simulink model "3.jmavsim_control_smc"  (R2023b)
settings: Solver=FixedStepAuto  StartTime=0.0  StopTime=inf  FixedStep=0.01  RelTol=1e-3  EnableMultiTasking=on
undefined symbols (not defined in the file): dev, Main, pwm_output0
libraries: simulink x19, px4uORBlib x3, sharedtransform x1, px4lib x1
settings Model: ExtModeTrigDuration=10  Creator=UAV2  LastModifiedBy=UAV2
settings SolverCC: PositivePriorityOrder=on
settings OptimizationCC: EnhancedBackFolding=on  PassReuseOutputArgsAs=Individual arguments  ZeroExternalMemoryAtStartup=off  ZeroInternalMemoryAtStartup=off  MaxStackSize=64  OptimizeBlockOrder=speed  DifferentSizesBufferReuse=on  EfficientTunableParamExpr=on
settings DebuggingCC: ParameterTunabilityLossMsg=error
settings HardwareCC: ProdBitPerPointer=32  ProdBitPerSizeT=32  ProdBitPerPtrDiffT=32  ProdLargestAtomicInteger=Long  ProdLargestAtomicFloat=Double  ProdWordSize=32  ProdLongLongMode=on  ProdHWDeviceType=ARM Compatible->ARM Cortex
settings SFSimCC: MATLABDynamicMemAlloc=off  SimTargetLang=C++
settings RTWCC: Description=Embedded Coder  SystemTargetFile=ert.tlc  HardwareBoard=PX4 Host Target  TemplateMakefile=ert_default_tmf  Toolchain=GNU Tools for PX4 Autopilots  PortableWordSizes=on  TargetLang=C++
settings CodeAppCC: ForceParamTrailComments=on  IgnoreCustomStorageClasses=off  OperatorAnnotations=on  SimulinkDataObjDesc=on  SFDataObjDesc=on  InsertBlockDesc=on
settings ERTTargetCC: ExtMode=on  ExtModeTransport=2  ExtModeStaticAlloc=on  ExtModeMexFile=ext_xcp  ExtModeMexArgs='127.0.0.1' 1 17725  ExtModeIntrfLevel=Level2 - Open

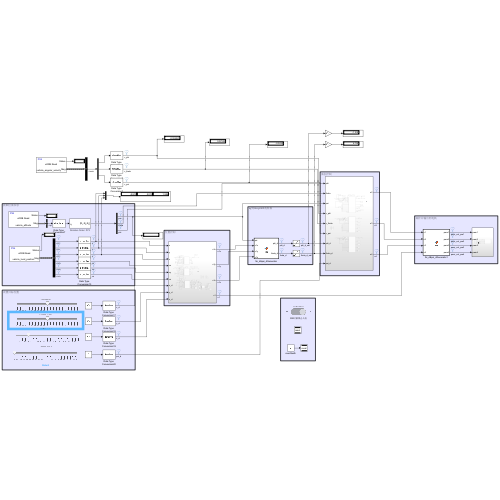
[thumbnail: Simulink's stored preview of the top-level diagram]
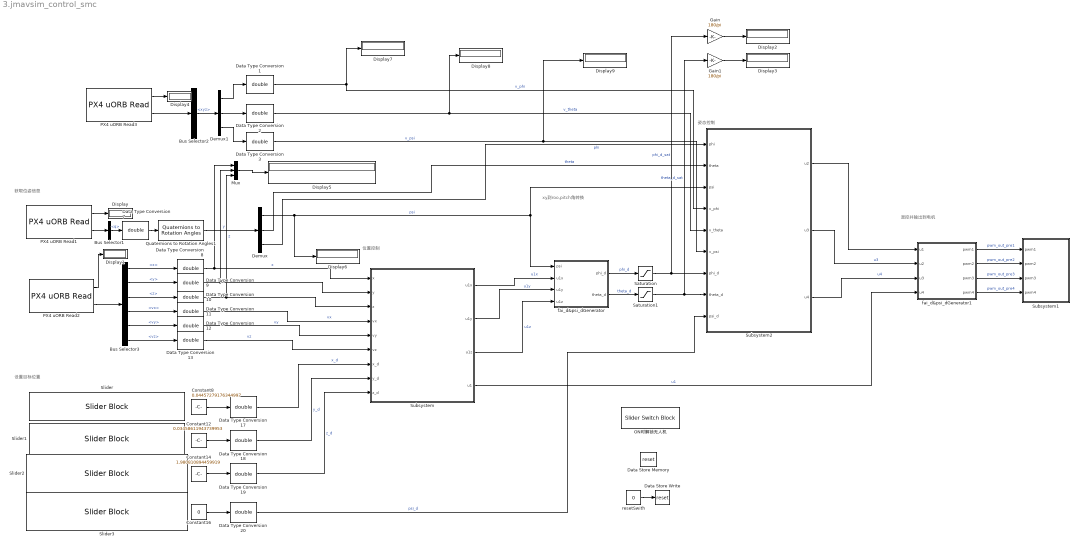
== system 3.jmavsim_control_smc ==
  note: 混控并输出到电机
  note: xy到roo,pitch角转换
  note: 姿态控制
  note: 位置控制
  note: 设置目标位置
  note: 获取位姿信息
  Bus Selector1 : BusSelector  OutputSignals=q
  Bus Selector2 : BusSelector  OutputSignals=xyz
  Bus Selector3 : BusSelector  OutputSignals=x,y,z,vx,vy,vz
  Constant12 : Constant  Value=0.03458611943739953
  Constant14 : Constant  Value=1.980810894459919
  Constant16 : Constant  Value=0
  Constant8 : Constant  Value=0.04457279176344997
  Data Store Memory : DataStoreMemory  DataStoreName=reset  WriteAfterWriteMsg=warning  ShowAdditionalParam=off  OutDataTypeStr=boolean
  Data Store Write : DataStoreWrite  DataStoreName=reset  IndexOptions=Index vector (dialog)  Indices=1  OutputSizes=1
  Data Type Conversion{1..3,7..13,17..20} (14 alike) : DataTypeConversion  OutDataTypeStr=double  SaturateOnIntegerOverflow=off  RndMeth=Floor
  Demux : Demux  Outputs=3
  Demux1 : Demux  Outputs=3
  Display{,1..9} (10 alike) : Display
      Display5 settings: Decimation=3
  Gain : Gain  Gain=180/pi
  Gain1 : Gain  Gain=180/pi
  Mux : Mux  Inputs=3
  ON时解锁无人机 : SliderSwitchBlock  Description=1时解锁无人机
      settings: Values={{'Off', 'On'}, [1 0]}
  PX4 uORB Read1 : px4uORBlib/PX4 uORB Read  uORBTopic=vehicle_attitude  selectInstance=vehicle_attitude_groundtruth  SampleTime=-1  BlockingMode=off  BlockTimeout=1e-3
  PX4 uORB Read2 : px4uORBlib/PX4 uORB Read  uORBTopic=vehicle_local_position  selectInstance=vehicle_local_position_groundtruth  SampleTime=-1  BlockingMode=off  BlockTimeout=1e-3
  PX4 uORB Read3 : px4uORBlib/PX4 uORB Read  uORBTopic=vehicle_angular_velocity  selectInstance=vehicle_angular_velocity  SampleTime=-1  BlockingMode=off  BlockTimeout=1e-3
  Quaternions to Rotation Angles1 : sharedtransform/Quaternions to Rotation Angles  rotationOrder=ZYX  aMode=aMode
  Saturation : Saturate
  Saturation1 : Saturate
  Slider : SliderBlock  ScaleMin=-10  ScaleMax=10
  Slider1 : SliderBlock  ScaleMin=-10  ScaleMax=10
  Slider2 : SliderBlock  ScaleMax=10
  Slider3 : SliderBlock  ScaleMax=2
  Subsystem : Subsystem
  Subsystem1 : Subsystem
  Subsystem2 : Subsystem
  fai_d&psi_dGenerator : MATLAB Function  TreatAsAtomicUnit=on
  fai_d&psi_dGenerator1 : MATLAB Function  TreatAsAtomicUnit=on
  resetSwith : Constant  Value=0  OutDataTypeStr=boolean
  wires:
  Constant8/1 -> Data Type Conversion17/1
  Quaternions to Rotation Angles1/1 -> Demux/1
  PX4 uORB Read1/1 -> Display/1
  PX4 uORB Read1/2 -> Bus Selector1/1
  Bus Selector1/1 -> Data Type Conversion7/1  "<q>"
  Data Type Conversion7/1 -> Quaternions to Rotation Angles1/1
  resetSwith/1 -> Data Store Write/1
  PX4 uORB Read2/2 -> Bus Selector3/1
  Bus Selector3/2 -> Data Type Conversion9/1  "<y>"
  Bus Selector3/3 -> Data Type Conversion10/1  "<z>"
  Bus Selector3/4 -> Data Type Conversion11/1  "<vx>"
  Bus Selector3/5 -> Data Type Conversion12/1  "<vy>"
  Bus Selector3/6 -> Data Type Conversion13/1  "<vz>"
  Bus Selector3/1 -> Data Type Conversion8/1  "<x>"
  PX4 uORB Read2/1 -> Display1/1
  Subsystem/2(u1y) -> fai_d&psi_dGenerator/3(u1y)  "u1y"
  fai_d&psi_dGenerator1/1(pwm1) -> Subsystem1/1(pwm1)  "pwm_out_pre1"
  fai_d&psi_dGenerator1/2(pwm2) -> Subsystem1/2(pwm2)  "pwm_out_pre2"
  fai_d&psi_dGenerator1/3(pwm3) -> Subsystem1/3(pwm3)  "pwm_out_pre3"
  fai_d&psi_dGenerator1/4(pwm4) -> Subsystem1/4(pwm4)  "pwm_out_pre4"
  Demux/1 -> Display6/1, fai_d&psi_dGenerator/1(psi), Subsystem2/3(psi)  "psi"
  Demux/2 -> Subsystem2/2(theta)  "theta"
  Demux/3 -> Subsystem2/1(phi)  "phi"
  Constant12/1 -> Data Type Conversion18/1
  Constant14/1 -> Data Type Conversion19/1
  Constant16/1 -> Data Type Conversion20/1
  Data Type Conversion20/1 -> Subsystem2/9(psi_d)  "psi_d"
  fai_d&psi_dGenerator/1(phi_d) -> Saturation/1  "phi_d"
  fai_d&psi_dGenerator/2(theta_d) -> Saturation1/1  "theta_d"
  Subsystem/3(u1z) -> fai_d&psi_dGenerator/4(u1z)  "u1z"
  Subsystem/4(u1) -> fai_d&psi_dGenerator1/4(u4)  "u1"
  Saturation1/1 -> Subsystem2/8(theta_d), Gain1/1  "theta_d_sat"
  Data Type Conversion8/1 -> Mux/1, Subsystem/1(x)  "x"
  Data Type Conversion9/1 -> Mux/2, Subsystem/2(y)  "y"
  Data Type Conversion10/1 -> Mux/3, Subsystem/3(z)  "z"
  Data Type Conversion12/1 -> Subsystem/5(vy)  "vy"
  Data Type Conversion13/1 -> Subsystem/6(vz)  "vz"
  Data Type Conversion17/1 -> Subsystem/7(x_d)  "x_d"
  Data Type Conversion18/1 -> Subsystem/8(y_d)  "y_d"
  Data Type Conversion19/1 -> Subsystem/9(z_d)  "z_d"
  Data Type Conversion11/1 -> Subsystem/4(vx)  "vx"
  Subsystem/1(u1x) -> fai_d&psi_dGenerator/2(u1x)  "u1x"
  Gain/1 -> Display2/1
  Gain1/1 -> Display3/1
  PX4 uORB Read3/2 -> Bus Selector2/1
  PX4 uORB Read3/1 -> Display4/1
  Data Type Conversion1/1 -> Display7/1, Subsystem2/4(v_phi)  "v_phi"
  Data Type Conversion2/1 -> Display8/1, Subsystem2/5(v_theta)  "v_theta"
  Data Type Conversion3/1 -> Display9/1, Subsystem2/6(v_psi)  "v_psi"
  Mux/1 -> Display5/1
  Bus Selector2/1 -> Demux1/1  "<xyz>"
  Demux1/1 -> Data Type Conversion1/1
  Demux1/2 -> Data Type Conversion2/1
  Demux1/3 -> Data Type Conversion3/1
  Saturation/1 -> Gain/1, Subsystem2/7(phi_d)  "phi_d_sat"
  Subsystem2/3(u4) -> fai_d&psi_dGenerator1/3(u3)  "u4"
  Subsystem2/1(u2) -> fai_d&psi_dGenerator1/1(u1)
  Subsystem2/2(u3) -> fai_d&psi_dGenerator1/2(u2)  "u3"

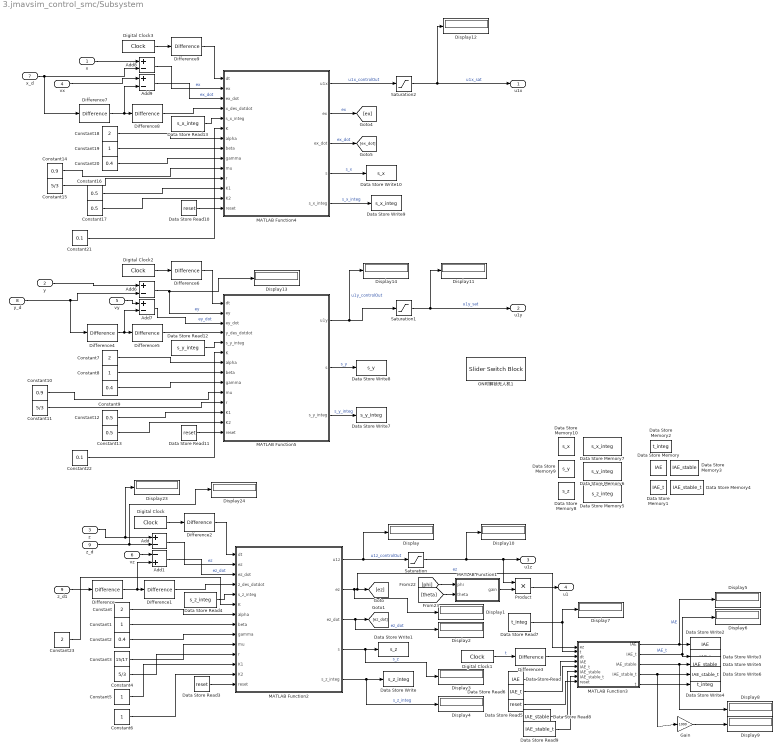
== system 3.jmavsim_control_smc/Subsystem ==
  x : Inport
  y : Inport  Port=2
  z : Inport  Port=3
  vx : Inport  Port=4
  vy : Inport  Port=5
  vz : Inport  Port=6
  x_d : Inport  Port=7
  y_d : Inport  Port=8
  z_d : Inport  Port=9
  Add{,6..9} (5 alike) : Sum  Inputs=+-
  Add1 : Sum  Inputs=-+
  Constant{,7,18,23} (4 alike) : Constant  Value=2
  Constant{1,5..6,8,19} (5 alike) : Constant
  Constant10 : Constant  Value=0.9
  Constant11 : Constant  Value=5/3
  Constant{12..13,16..17} (4 alike) : Constant  Value=0.5
  Constant14 : Constant  Value=0.9
  Constant15 : Constant  Value=5/3
  Constant2 : Constant  Value=0.4
  Constant20 : Constant  Value=0.4
  Constant21 : Constant  Value=0.1
  Constant22 : Constant  Value=0.1
  Constant3 : Constant  Value=15/17
  Constant4 : Constant  Value=5/3
  Constant9 : Constant  Value=0.4
  Data Store Memory : DataStoreMemory  DataStoreName=IAE  WriteAfterWriteMsg=warning  ShowAdditionalParam=off
  Data Store Memory1 : DataStoreMemory  DataStoreName=IAE_t  WriteAfterWriteMsg=warning  ShowAdditionalParam=off
  Data Store Memory10 : DataStoreMemory  DataStoreName=s_x  WriteAfterWriteMsg=warning  ShowAdditionalParam=off  OutDataTypeStr=double
  Data Store Memory2 : DataStoreMemory  DataStoreName=t_integ  WriteAfterWriteMsg=warning  ShowAdditionalParam=off
  Data Store Memory3 : DataStoreMemory  DataStoreName=IAE_stable  WriteAfterWriteMsg=warning  ShowAdditionalParam=off
  Data Store Memory4 : DataStoreMemory  DataStoreName=IAE_stable_t  WriteAfterWriteMsg=warning  ShowAdditionalParam=off
  Data Store Memory5 : DataStoreMemory  DataStoreName=s_z_integ  WriteAfterWriteMsg=warning  ShowAdditionalParam=off  OutDataTypeStr=double
  Data Store Memory6 : DataStoreMemory  DataStoreName=s_y_integ  WriteAfterWriteMsg=warning  ShowAdditionalParam=off  OutDataTypeStr=double
  Data Store Memory7 : DataStoreMemory  DataStoreName=s_x_integ  WriteAfterWriteMsg=warning  ShowAdditionalParam=off  OutDataTypeStr=double
  Data Store Memory8 : DataStoreMemory  DataStoreName=s_z  WriteAfterWriteMsg=warning  ShowAdditionalParam=off  OutDataTypeStr=double
  Data Store Memory9 : DataStoreMemory  DataStoreName=s_y  WriteAfterWriteMsg=warning  ShowAdditionalParam=off  OutDataTypeStr=double
  Data Store Read : DataStoreRead  DataStoreName=IAE  IndexOptions=Index vector (dialog)  Indices=1  OutputSizes=1
  Data Store Read{3,5,10..11} (4 alike) : DataStoreRead  DataStoreName=reset  IndexOptions=Index vector (dialog)  Indices=1  OutputSizes=1
  Data Store Read12 : DataStoreRead  DataStoreName=s_y_integ  IndexOptions=Index vector (dialog)  Indices=1  OutputSizes=1
  Data Store Read13 : DataStoreRead  DataStoreName=s_x_integ  IndexOptions=Index vector (dialog)  Indices=1  OutputSizes=1
  Data Store Read4 : DataStoreRead  DataStoreName=s_z_integ  IndexOptions=Index vector (dialog)  Indices=1  OutputSizes=1
  Data Store Read6 : DataStoreRead  DataStoreName=IAE_t  IndexOptions=Index vector (dialog)  Indices=1  OutputSizes=1
  Data Store Read7 : DataStoreRead  DataStoreName=t_integ  IndexOptions=Index vector (dialog)  Indices=1  OutputSizes=1
  Data Store Read8 : DataStoreRead  DataStoreName=IAE_stable  IndexOptions=Index vector (dialog)  Indices=1  OutputSizes=1
  Data Store Read9 : DataStoreRead  DataStoreName=IAE_stable_t  IndexOptions=Index vector (dialog)  Indices=1  OutputSizes=1
  Data Store Write : DataStoreWrite  DataStoreName=s_z_integ  IndexOptions=Index vector (dialog)  Indices=1  OutputSizes=1
  Data Store Write1 : DataStoreWrite  DataStoreName=s_z  IndexOptions=Index vector (dialog)  Indices=1  OutputSizes=1
  Data Store Write10 : DataStoreWrite  DataStoreName=s_x  IndexOptions=Index vector (dialog)  Indices=1  OutputSizes=1
  Data Store Write2 : DataStoreWrite  DataStoreName=IAE  IndexOptions=Index vector (dialog)  Indices=1  OutputSizes=1
  Data Store Write3 : DataStoreWrite  DataStoreName=IAE_t  IndexOptions=Index vector (dialog)  Indices=1  OutputSizes=1
  Data Store Write4 : DataStoreWrite  DataStoreName=t_integ  IndexOptions=Index vector (dialog)  Indices=1  OutputSizes=1
  Data Store Write5 : DataStoreWrite  DataStoreName=IAE_stable  IndexOptions=Index vector (dialog)  Indices=1  OutputSizes=1
  Data Store Write6 : DataStoreWrite  DataStoreName=IAE_stable_t  IndexOptions=Index vector (dialog)  Indices=1  OutputSizes=1
  Data Store Write7 : DataStoreWrite  DataStoreName=s_y_integ  IndexOptions=Index vector (dialog)  Indices=1  OutputSizes=1
  Data Store Write8 : DataStoreWrite  DataStoreName=s_y  IndexOptions=Index vector (dialog)  Indices=1  OutputSizes=1
  Data Store Write9 : DataStoreWrite  DataStoreName=s_x_integ  IndexOptions=Index vector (dialog)  Indices=1  OutputSizes=1
  Difference{,1..9} (10 alike) : simulink/Discrete/Difference  ICPrevInput=0.0  OutMin=[]  OutMax=[]  OutDataType=fixdt(1, 16)  OutScaling=2^-10  DoSatur=off
  Digital Clock{,1..3} (4 alike) : DigitalClock  SampleTime=0.01
  Display{,1..14,23..24} (17 alike) : Display
  Gain : Gain  Gain=1000
  MATLAB Function1 : MATLAB Function  TreatAsAtomicUnit=on
  MATLAB Function2 : MATLAB Function  TreatAsAtomicUnit=on
  MATLAB Function3 : MATLAB Function  TreatAsAtomicUnit=on
  MATLAB Function4 : MATLAB Function  TreatAsAtomicUnit=on
  MATLAB Function5 : MATLAB Function  TreatAsAtomicUnit=on
  ON时解锁无人机1 : SliderSwitchBlock  Description=1时解锁无人机
      settings: Values={{'Off', 'On'}, [1 0]}
  Product : Product
  Saturation : Saturate  UpperLimit=1  LowerLimit=0
  Saturation1 : Saturate
  Saturation2 : Saturate  UpperLimit=1  LowerLimit=-1
  z_d1 : InportShadow  Port=9
  u1x : Outport
  u1y : Outport  Port=2
  u1z : Outport  Port=3
  u1 : Outport  Port=4
  wires:
  [phi] -> MATLAB Function1/1(phi)
  Product/1 -> u1/1
  [theta] -> MATLAB Function1/2(theta)
  MATLAB Function1/1(gain) -> Product/2
  MATLAB Function2/1(u1z) -> Display/1, Saturation/1  "u1z_controlOut"
  z_d1/1 -> Difference/1
  Difference/1 -> Add1/2, Difference1/1
  Difference1/1 -> MATLAB Function2/4(z_des_dotdot)
  Data Store Read3/1 -> MATLAB Function2/14(reset)
  Data Store Read4/1 -> MATLAB Function2/5("s_z_integ ")
  Digital Clock/1 -> Difference2/1
  Difference2/1 -> MATLAB Function2/1(dt)
  MATLAB Function2/4(s) -> Data Store Write1/1, Display3/1  "s_z"
  MATLAB Function2/5(s_z_integ) -> Display4/1, Data Store Write/1  "s_z_integ"
  MATLAB Function2/2(ez) -> MATLAB Function3/1(ez), [ez], Display1/1  "ez"
  MATLAB Function2/3(ez_dot) -> [ez_dot], Display2/1  "ez_dot"
  Saturation/1 -> Display10/1, u1z/1, Product/1
  Add/1 -> MATLAB Function2/2("ez ")  "ez"
  z_d/1 -> Display24/1, Add/2
  vz/1 -> Add1/1
  Add1/1 -> MATLAB Function2/3("ez_dot ")  "ez_dot"
  Constant/1 -> MATLAB Function2/7(alpha)
  Constant1/1 -> MATLAB Function2/8(beta)
  Constant2/1 -> MATLAB Function2/9(gamma)
  Constant3/1 -> MATLAB Function2/10(mu)
  Constant4/1 -> MATLAB Function2/11(r)
  Constant5/1 -> MATLAB Function2/12(K1)
  Constant6/1 -> MATLAB Function2/13(K2)
  Data Store Read5/1 -> MATLAB Function3/8(reset)
  Difference3/1 -> MATLAB Function3/3(dt)
  MATLAB Function3/1(IAE) -> Display5/1, Data Store Write2/1  "IAE"
  MATLAB Function3/2(IAE_t) -> Display6/1, Data Store Write3/1  "IAE_t"
  Digital Clock1/1 -> Difference3/1  "t"
  Data Store Read/1 -> MATLAB Function3/4("IAE ")
  Data Store Read6/1 -> MATLAB Function3/5("IAE_t ")
  Data Store Read7/1 -> MATLAB Function3/2("t "), Display7/1
  MATLAB Function3/5(t) -> Data Store Write4/1
  MATLAB Function3/3(IAE_stable) -> Display8/1, Data Store Write5/1
  MATLAB Function3/4(IAE_stable_t) -> Gain/1, Data Store Write6/1
  Data Store Read8/1 -> MATLAB Function3/6("IAE_stable ")
  Data Store Read9/1 -> MATLAB Function3/7("IAE_stable_t ")
  Gain/1 -> Display9/1
  Constant7/1 -> MATLAB Function5/7(alpha)
  Constant10/1 -> MATLAB Function5/10(mu)
  Constant13/1 -> MATLAB Function5/13(K2)
  Constant12/1 -> MATLAB Function5/12(K1)
  Add7/1 -> MATLAB Function5/3(ey_dot)  "ey_dot"
  Constant11/1 -> MATLAB Function5/11(r)
  Difference4/1 -> Add7/2, Difference5/1
  Data Store Read12/1 -> MATLAB Function5/5("s_y_integ ")
  Constant9/1 -> MATLAB Function5/9(gamma)
  MATLAB Function5/1(u1y) -> Display14/1, Saturation1/1  "u1y_controlOut"
  Constant8/1 -> MATLAB Function5/8(beta)
  Data Store Read11/1 -> MATLAB Function5/14(reset)
  MATLAB Function5/3(s_y_integ) -> Data Store Write7/1  "s_y_integ"
  Difference5/1 -> MATLAB Function5/4(y_des_dotdot)
  Digital Clock2/1 -> Difference6/1
  vy/1 -> Add7/1
  Add6/1 -> MATLAB Function5/2(ey), Display13/1  "ey"
  Saturation1/1 -> Display11/1, u1y/1  "u1y_sat"
  Difference6/1 -> MATLAB Function5/1(dt)
  y/1 -> Add6/1
  MATLAB Function5/2(s) -> Data Store Write8/1  "s_y"
  Difference8/1 -> MATLAB Function4/4(x_des_dotdot)
  Data Store Read10/1 -> MATLAB Function4/14(reset)
  Constant20/1 -> MATLAB Function4/9(gamma)
  MATLAB Function4/1(u1x) -> Saturation2/1  "u1x_controlOut"
  Constant19/1 -> MATLAB Function4/8(beta)
  Data Store Read13/1 -> MATLAB Function4/5("s_x_integ ")
  Difference7/1 -> Add9/2, Difference8/1
  Add9/1 -> MATLAB Function4/3("ex_dot ")  "ex_dot"
  Constant15/1 -> MATLAB Function4/11(r)
  Constant17/1 -> MATLAB Function4/13(K2)
  Constant14/1 -> MATLAB Function4/10(mu)
  Constant16/1 -> MATLAB Function4/12(K1)
  Constant18/1 -> MATLAB Function4/7(alpha)
  MATLAB Function4/2(ex) -> [ex]  "ex"
  Saturation2/1 -> Display12/1, u1x/1  "u1x_sat"
  MATLAB Function4/5(s_x_integ) -> Data Store Write9/1  "s_x_integ"
  Digital Clock3/1 -> Difference9/1
  Add8/1 -> MATLAB Function4/2("ex ")  "ex"
  Difference9/1 -> MATLAB Function4/1(dt)
  MATLAB Function4/3(ex_dot) -> [ex_dot]  "ex_dot"
  MATLAB Function4/4(s) -> Data Store Write10/1  "s_x"
  z/1 -> Display23/1, Add/1
  x/1 -> Add8/1
  vx/1 -> Add9/1
  x_d/1 -> Difference7/1, Add8/2
  Constant21/1 -> MATLAB Function4/6(K)
  Constant22/1 -> MATLAB Function5/6(K)
  Constant23/1 -> MATLAB Function2/6(K)
  y_d/1 -> Difference4/1, Add6/2

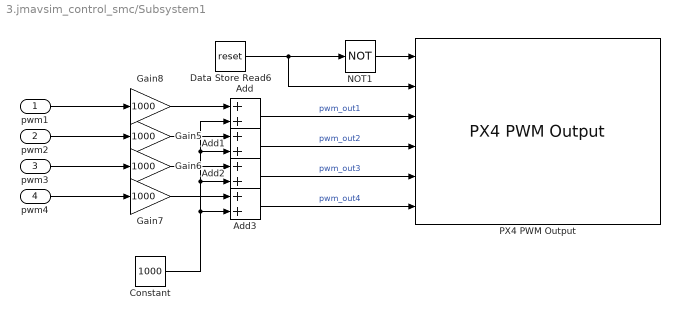
== system 3.jmavsim_control_smc/Subsystem1 ==
  pwm1 : Inport
  pwm2 : Inport  Port=2
  pwm3 : Inport  Port=3
  pwm4 : Inport  Port=4
  Add{,1..3} (4 alike) : Sum  OutDataTypeStr=uint16
  Constant : Constant  Value=1000
  Data Store Read6 : DataStoreRead  DataStoreName=reset  IndexOptions=Index vector (dialog)  Indices=1  OutputSizes=1
  Gain{5..8} (4 alike) : Gain  Gain=1000  OutDataTypeStr=uint16
  NOT1 : Logic  Operator=NOT  IconShape=distinctive  AllPortsSameDT=off  OutDataTypeStr=boolean
  PX4 PWM Output : px4lib/PX4 PWM Output  pwmDevice=Main (/dev/pwm_output0)  pwmChannel1_=on  pwmChannel2_=on  pwmChannel3_=on  pwmChannel4_=on  pwmChannel5_=off  pwmChannel6_=off  pwmChannel7_=off  pwmChannel8_=off  forceTerminateFailsafe=off  outputErrorStatus=off
  wires:
  NOT1/1 -> PX4 PWM Output/1
  Add3/1 -> PX4 PWM Output/6  "pwm_out4"
  Data Store Read6/1 -> PX4 PWM Output/2, NOT1/1
  Add/1 -> PX4 PWM Output/3  "pwm_out1"
  Add1/1 -> PX4 PWM Output/4  "pwm_out2"
  pwm3/1 -> Gain6/1
  pwm1/1 -> Gain8/1
  pwm2/1 -> Gain5/1
  pwm4/1 -> Gain7/1
  Add2/1 -> PX4 PWM Output/5  "pwm_out3"
  Gain8/1 -> Add/1
  Constant/1 -> Add3/2, Add2/2, Add1/2, Add/2
  Gain5/1 -> Add1/1
  Gain7/1 -> Add3/1
  Gain6/1 -> Add2/1

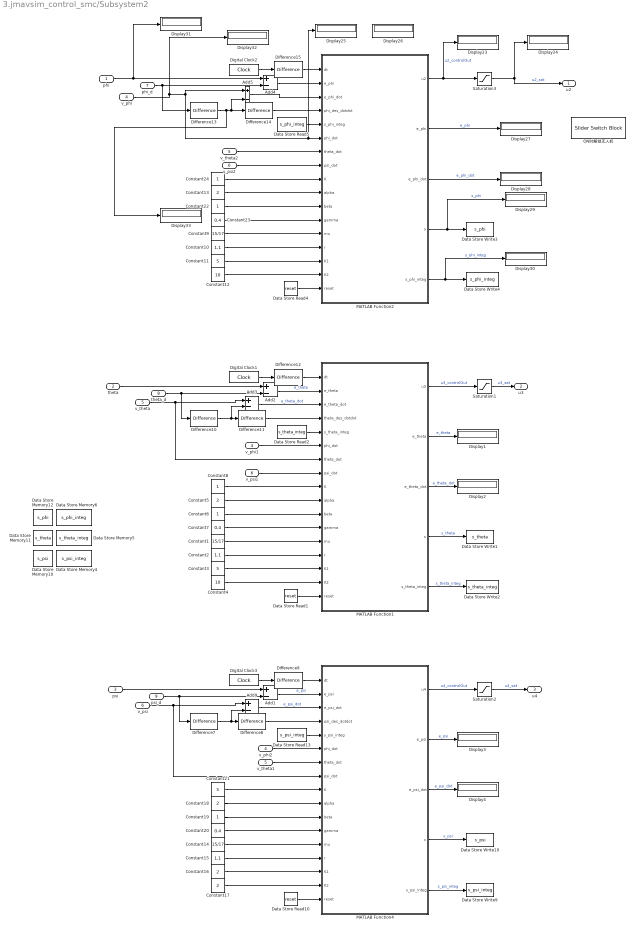
== system 3.jmavsim_control_smc/Subsystem2 ==
  phi : Inport
  theta : Inport  Port=2
  psi : Inport  Port=3
  v_phi : Inport  Port=4
  v_theta : Inport  Port=5
  v_psi : Inport  Port=6
  phi_d : Inport  Port=7
  theta_d : Inport  Port=8
  psi_d : Inport  Port=9
  Add{1..5,9} (6 alike) : Sum  Inputs=+-
  Constant1 : Constant  Value=15/17
  Constant10 : Constant  Value=1.1
  Constant11 : Constant  Value=5
  Constant12 : Constant  Value=10
  Constant{5,13,16..18} (5 alike) : Constant  Value=2
  Constant14 : Constant  Value=15/17
  Constant15 : Constant  Value=1.1
  Constant{6,8,19,22,24} (5 alike) : Constant
  Constant2 : Constant  Value=1.1
  Constant20 : Constant  Value=0.4
  Constant21 : Constant  Value=5
  Constant23 : Constant  Value=0.4
  Constant3 : Constant  Value=5
  Constant4 : Constant  Value=10
  Constant7 : Constant  Value=0.4
  Constant9 : Constant  Value=15/17
  Data Store Memory10 : DataStoreMemory  DataStoreName=s_psi  WriteAfterWriteMsg=warning  ShowAdditionalParam=off  OutDataTypeStr=double
  Data Store Memory11 : DataStoreMemory  DataStoreName=s_theta  WriteAfterWriteMsg=warning  ShowAdditionalParam=off  OutDataTypeStr=double
  Data Store Memory12 : DataStoreMemory  DataStoreName=s_phi  WriteAfterWriteMsg=warning  ShowAdditionalParam=off  OutDataTypeStr=double
  Data Store Memory4 : DataStoreMemory  DataStoreName=s_psi_integ  WriteAfterWriteMsg=warning  ShowAdditionalParam=off  OutDataTypeStr=double
  Data Store Memory5 : DataStoreMemory  DataStoreName=s_theta_integ  WriteAfterWriteMsg=warning  ShowAdditionalParam=off  OutDataTypeStr=double
  Data Store Memory6 : DataStoreMemory  DataStoreName=s_phi_integ  WriteAfterWriteMsg=warning  ShowAdditionalParam=off  OutDataTypeStr=double
  Data Store Read1 : DataStoreRead  DataStoreName=reset  IndexOptions=Index vector (dialog)  Indices=1  OutputSizes=1
  Data Store Read10 : DataStoreRead  DataStoreName=reset  IndexOptions=Index vector (dialog)  Indices=1  OutputSizes=1
  Data Store Read13 : DataStoreRead  DataStoreName=s_psi_integ  IndexOptions=Index vector (dialog)  Indices=1  OutputSizes=1
  Data Store Read2 : DataStoreRead  DataStoreName=s_theta_integ  IndexOptions=Index vector (dialog)  Indices=1  OutputSizes=1
  Data Store Read4 : DataStoreRead  DataStoreName=reset  IndexOptions=Index vector (dialog)  Indices=1  OutputSizes=1
  Data Store Read5 : DataStoreRead  DataStoreName=s_phi_integ  IndexOptions=Index vector (dialog)  Indices=1  OutputSizes=1
  Data Store Write1 : DataStoreWrite  DataStoreName=s_theta  IndexOptions=Index vector (dialog)  Indices=1  OutputSizes=1
  Data Store Write10 : DataStoreWrite  DataStoreName=s_psi  IndexOptions=Index vector (dialog)  Indices=1  OutputSizes=1
  Data Store Write2 : DataStoreWrite  DataStoreName=s_theta_integ  IndexOptions=Index vector (dialog)  Indices=1  OutputSizes=1
  Data Store Write3 : DataStoreWrite  DataStoreName=s_phi  IndexOptions=Index vector (dialog)  Indices=1  OutputSizes=1
  Data Store Write4 : DataStoreWrite  DataStoreName=s_phi_integ  IndexOptions=Index vector (dialog)  Indices=1  OutputSizes=1
  Data Store Write9 : DataStoreWrite  DataStoreName=s_psi_integ  IndexOptions=Index vector (dialog)  Indices=1  OutputSizes=1
  Difference{7..15} (9 alike) : simulink/Discrete/Difference  ICPrevInput=0.0  OutMin=[]  OutMax=[]  OutDataType=fixdt(1, 16)  OutScaling=2^-10  DoSatur=off
  Digital Clock1 : DigitalClock  SampleTime=0.01
  Digital Clock2 : DigitalClock  SampleTime=0.01
  Digital Clock3 : DigitalClock  SampleTime=0.01
  Display{1..4,23..33} (15 alike) : Display
  MATLAB Function1 : MATLAB Function  TreatAsAtomicUnit=on
  MATLAB Function2 : MATLAB Function  TreatAsAtomicUnit=on
  MATLAB Function4 : MATLAB Function  TreatAsAtomicUnit=on
  ON时解锁无人机 : SliderSwitchBlock  Description=1时解锁无人机
      settings: Values={{'Off', 'On'}, [1 0]}
  Saturation1 : Saturate  UpperLimit=0.1  LowerLimit=-0.1
  Saturation2 : Saturate  UpperLimit=0.2  LowerLimit=-0.2
  Saturation3 : Saturate  UpperLimit=0.1  LowerLimit=-0.1
  v_phi1 : InportShadow  Port=4
  v_phi2 : InportShadow  Port=4
  v_psi1 : InportShadow  Port=6
  v_psi2 : InportShadow  Port=6
  v_theta1 : InportShadow  Port=5
  v_theta2 : InportShadow  Port=5
  u2 : Outport
  u3 : Outport  Port=2
  u4 : Outport  Port=3
  wires:
  Data Store Read10/1 -> MATLAB Function4/17(reset)
  Data Store Read13/1 -> MATLAB Function4/5("s_psi_integ ")
  MATLAB Function4/5(s_psi_integ) -> Data Store Write9/1  "s_psi_integ"
  Saturation2/1 -> u4/1  "u4_sat"
  Constant18/1 -> MATLAB Function4/10(alpha)
  Constant17/1 -> MATLAB Function4/16(K2)
  Constant15/1 -> MATLAB Function4/14(r)
  Add9/1 -> MATLAB Function4/3("e_psi_dot ")  "e_psi_dot"
  Difference7/1 -> Add9/2, Difference8/1
  Constant19/1 -> MATLAB Function4/11(beta)
  Difference8/1 -> MATLAB Function4/4(psi_des_dotdot)
  Difference9/1 -> MATLAB Function4/1(dt)
  MATLAB Function4/4(s) -> Data Store Write10/1  "s_psi"
  MATLAB Function4/2(e_psi) -> Display3/1  "e_psi"
  MATLAB Function4/3(e_psi_dot) -> Display4/1  "e_psi_dot"
  MATLAB Function4/1(u4) -> Saturation2/1  "u4_controlOut"
  Digital Clock3/1 -> Difference9/1
  Constant14/1 -> MATLAB Function4/13(mu)
  Constant20/1 -> MATLAB Function4/12(gamma)
  Constant16/1 -> MATLAB Function4/15(K1)
  Constant21/1 -> MATLAB Function4/9(K)
  psi/1 -> Add1/1
  Add1/1 -> MATLAB Function4/2("e_psi ")  "e_psi"
  Constant3/1 -> MATLAB Function1/15(K1)
  Constant4/1 -> MATLAB Function1/16(K2)
  MATLAB Function1/3(e_theta_dot) -> Display2/1  "e_theta_dot"
  Difference12/1 -> MATLAB Function1/1(dt)
  Digital Clock1/1 -> Difference12/1
  Difference11/1 -> MATLAB Function1/4(theta_des_dotdot)
  Constant8/1 -> MATLAB Function1/9(K)
  MATLAB Function1/1(u3) -> Saturation1/1  "u3_controlOut"
  MATLAB Function1/2(e_theta) -> Display1/1  "e_theta"
  Constant7/1 -> MATLAB Function1/12(gamma)
  Constant1/1 -> MATLAB Function1/13(mu)
  Data Store Read2/1 -> MATLAB Function1/5("s_theta_integ ")
  MATLAB Function1/4(s) -> Data Store Write1/1  "s_theta"
  Difference10/1 -> Add3/2, Difference11/1
  Constant5/1 -> MATLAB Function1/10(alpha)
  Data Store Read1/1 -> MATLAB Function1/17(reset)
  Add2/1 -> MATLAB Function1/2("e_theta ")  "e_theta"
  Add3/1 -> MATLAB Function1/3("e_theta_dot ")  "e_theta_dot"
  MATLAB Function1/5(s_theta_integ) -> Data Store Write2/1  "s_theta_integ"
  theta/1 -> Add2/1
  Constant2/1 -> MATLAB Function1/14(r)
  Constant6/1 -> MATLAB Function1/11(beta)
  Constant10/1 -> MATLAB Function2/14(r)
  Saturation3/1 -> u2/1, Display24/1  "u2_sat"
  phi/1 -> Display31/1, Add4/1
  Constant13/1 -> MATLAB Function2/10(alpha)
  Difference13/1 -> Display33/1, Add5/2, Difference14/1
  Data Store Read4/1 -> MATLAB Function2/17(reset)
  Constant23/1 -> MATLAB Function2/12(gamma)
  MATLAB Function2/2(e_phi) -> Display27/1  "e_phi"
  MATLAB Function2/1(u2) -> Display23/1, Saturation3/1  "u2_controlOut"
  Constant22/1 -> MATLAB Function2/11(beta)
  Data Store Read5/1 -> MATLAB Function2/5("s_phi_integ ")
  Constant9/1 -> MATLAB Function2/13(mu)
  Constant24/1 -> MATLAB Function2/9(K)
  Difference14/1 -> MATLAB Function2/4(phi_des_dotdot)
  Digital Clock2/1 -> Difference15/1
  Difference15/1 -> MATLAB Function2/1(dt)
  MATLAB Function2/3(e_phi_dot) -> Display28/1  "e_phi_dot"
  Add5/1 -> MATLAB Function2/3("e_phi_dot ")
  Constant11/1 -> MATLAB Function2/15(K1)
  MATLAB Function2/4(s) -> Display29/1, Data Store Write3/1  "s_phi"
  Add4/1 -> MATLAB Function2/2("e_phi ")
  MATLAB Function2/5(s_phi_integ) -> Display30/1, Data Store Write4/1  "s_phi_integ"
  Constant12/1 -> MATLAB Function2/16(K2)
  v_phi/1 -> Display32/1, Add5/1, Display25/1, MATLAB Function2/6(phi_dot)
  v_theta/1 -> Add3/1, MATLAB Function1/7(theta_dot)
  v_psi/1 -> Add9/1, MATLAB Function4/8(psi_dot)
  v_phi1/1 -> MATLAB Function1/6(phi_dot)
  v_theta2/1 -> MATLAB Function2/7(theta_dot)
  v_psi2/1 -> MATLAB Function2/8(psi_dot)
  v_psi1/1 -> MATLAB Function1/8(psi_dot)
  v_phi2/1 -> MATLAB Function4/6(phi_dot)
  v_theta1/1 -> MATLAB Function4/7(theta_dot)
  Saturation1/1 -> u3/1  "u3_sat"
  psi_d/1 -> Difference7/1, Add1/2
  theta_d/1 -> Add2/2, Difference10/1
  phi_d/1 -> Add4/2, Difference13/1

== matlab function 3.jmavsim_control_smc/Subsystem/MATLAB Function5 ==
  data: dt input; ey input double; u1y output double; ey_dot input double; y_des_dotdot input; s_y_integ input; K input; alpha input; beta input; gamma input; mu input; r input; K1 input; K2 input; reset input; s output; s_y_integ output
function [u1y, s, s_y_integ] = u1yfcn(dt, ey, ey_dot, y_des_dotdot,...
                    s_y_integ, K, alpha, beta, gamma, mu, r, K1, K2, reset)

if (reset == 1); s_y_integ = 0; end
m = 0.8; g = 9.80665; %Ix = 0.005; Iy = 0.005; Iz = 0.009; L = 0.33 / 2;
Ky = 0;

% alpha = 2;beta = 1;gamma = 0.4;
% mu = 15/17;r = 5/3;
% K1 = 1;K2 = 1;

s = alpha * ey +  (beta * sign(ey_dot) * (abs(ey_dot)) ^ mu) + (gamma * sign(ey) * (abs(ey)) ^ r);
s_y_integ = s_y_integ + K2 * sign(s) * dt;

u1y = -m*(- Ky/m*ey_dot - y_des_dotdot + alpha/(beta*mu)*sign(ey_dot) * (abs(ey_dot))^(2-mu)...
    + gamma*r/(beta*mu)*(sign(ey) * (abs(ey))^(r-1))* sign(ey_dot) * (abs(ey_dot))^(2-mu) + K1*(abs(s))^(1/2)*sign(s)...
    + s_y_integ);

u1y = u1y * K;

== matlab function 3.jmavsim_control_smc/Subsystem2/MATLAB Function4 ==
  data: dt input; e_psi input double; u4 output double; e_psi output; e_psi_dot output; e_psi_dot input double; psi_des_dotdot input; s_psi_integ input; phi_dot input; theta_dot input; psi_dot input; K input; alpha input; beta input; gamma input; mu input; r input; K1 input; K2 input; reset input; s output; s_psi_integ output
function [u4, e_psi, e_psi_dot, s, s_psi_integ] = u4fcn(dt, e_psi, e_psi_dot, psi_des_dotdot,...
                    s_psi_integ, phi_dot, theta_dot, psi_dot, K,alpha, beta, gamma, mu, r, K1, K2, reset)

if (reset == 1); s_psi_integ = 0; end
m = 0.8; g = 9.80665; Ix = 0.005; Iy = 0.005; Iz = 0.009; L = 0.33 / 2;
Kpsi = 0;

% alpha = 2;beta = 1;gamma = 0.4;
% mu = 15/17;r = 5/3;
% K1 = 1;K2 = 1;

s = alpha * e_psi +  real(beta * sign(e_psi_dot) * (abs(e_psi_dot)) ^ mu) + real(gamma * sign(e_psi) * (abs(e_psi)) ^ r);
s_psi_integ = s_psi_integ + K2 * sign(s) * dt;

u4 = -Iz*((Ix-Iy)/Iz*phi_dot*theta_dot - Kpsi/Iz*psi_dot - psi_des_dotdot + alpha/(beta*mu)*sign(e_psi_dot) * (abs(e_psi_dot))^(2-mu)...
    + gamma*r/(beta*mu)*(sign(e_psi) * (abs(e_psi))^(r-1))* sign(e_psi_dot) * (abs(e_psi_dot))^(2-mu) + K1*(abs(s))^(1/2)*sign(s)...
    + s_psi_integ);
u4 = u4 * K;

== matlab function 3.jmavsim_control_smc/fai_d&psi_dGenerator ==
  data: psi input double; phi_d output double; u1x input double; u1y input double; u1z input double; theta_d output double
function [phi_d, theta_d] = fcn(psi, u1x, u1y, u1z)

% fai_d = atan((y_d - y)/(x_d - x));
% theta_d = atan((z_d - z)/(((x_d - x)^2 + (y_d - y)^2)^(1/2)));
phi_d = -1 * atan((u1x * sin(psi) - u1y * cos(psi)) / u1z );
theta_d = -1 * atan((u1x * cos(psi) + u1y * sin(psi)) * cos(phi_d) / u1z );

== matlab function 3.jmavsim_control_smc/Subsystem/MATLAB Function1 ==
  data: phi input double; gain output double; theta input double
function gain = fcn(phi, theta)

gain = 1/(cos(phi) * cos(theta));

== matlab function 3.jmavsim_control_smc/Subsystem2/MATLAB Function1 ==
  data: dt input; e_theta input double; u3 output double; e_theta output; e_theta_dot output; e_theta_dot input double; theta_des_dotdot input; s_theta_integ input; phi_dot input; theta_dot input; psi_dot input; K input; alpha input; beta input; gamma input; mu input; r input; K1 input; K2 input; reset input; s output; s_theta_integ output
function [u3, e_theta, e_theta_dot, s, s_theta_integ] = u3fcn(dt, e_theta, e_theta_dot, theta_des_dotdot,...
                    s_theta_integ, phi_dot, theta_dot, psi_dot, K,alpha, beta, gamma, mu, r, K1, K2, reset)

if (reset == 1); s_theta_integ = 0; end
m = 0.8; g = 9.80665; Ix = 0.005; Iy = 0.005; Iz = 0.009; L = 0.33 / 2;
Ktheta = 0;

% alpha = 2;beta = 1;gamma = 0.4;
% mu = 15/17;r = 5/3;
% K1 = 1;K2 = 1;
K2 = (K1^2)/2;

s = alpha * e_theta +  (beta * sign(e_theta_dot) * (abs(e_theta_dot)) ^ mu) + (gamma * sign(e_theta) * (abs(e_theta)) ^ r);
s_theta_integ = s_theta_integ + K2 * sign(s) * dt;

u3 = -Iy*((Iz-Ix)/Iy*phi_dot*psi_dot - Ktheta/Iy*theta_dot - theta_des_dotdot + alpha/(beta*mu)*sign(e_theta_dot) * (abs(e_theta_dot))^(2-mu)...
    + gamma*r/(beta*mu)*(sign(e_theta) * (abs(e_theta))^(r-1))* sign(e_theta_dot) * (abs(e_theta_dot))^(2-mu) + K1*(abs(s))^(1/2)*sign(s)...
    + s_theta_integ);
u3 = u3 * K;

== matlab function 3.jmavsim_control_smc/Subsystem2/MATLAB Function2 ==
  data: dt input; e_phi input double; u2 output double; e_phi output; e_phi_dot output; e_phi_dot input double; phi_des_dotdot input; s_phi_integ input; phi_dot input; theta_dot input; psi_dot input; K input; alpha input; beta input; gamma input; mu input; r input; K1 input; K2 input; reset input; s output; s_phi_integ output
function [u2, e_phi, e_phi_dot, s, s_phi_integ] = u2fcn(dt, e_phi, e_phi_dot, phi_des_dotdot,...
                    s_phi_integ, phi_dot, theta_dot, psi_dot, K,alpha, beta, gamma, mu, r, K1, K2, reset)

if (reset == 1); s_phi_integ = 0; end
m = 0.8; g = 9.80665; Ix = 0.005; Iy = 0.005; Iz = 0.009; L = 0.33 / 2;
Kphi = 0;

% alpha = 2;beta = 1;gamma = 0.4;
% mu = 15/17;r = 5/3;
% K1 = 1;K2 = 1;
K2 = (K1^2)/2;

s = alpha * e_phi +  (beta * sign(e_phi_dot) * (abs(e_phi_dot)) ^ mu) + (gamma * sign(e_phi) * (abs(e_phi)) ^ r);
s_phi_integ = s_phi_integ + K2 * sign(s) * dt;

u2 = -Ix*((Iy-Iz)/Ix*theta_dot*psi_dot - Kphi/Ix*phi_dot - phi_des_dotdot + alpha/(beta*mu)*sign(e_phi_dot) * (abs(e_phi_dot))^(2-mu)...
    + gamma*r/(beta*mu)*(sign(e_phi) * (abs(e_phi))^(r-1))* sign(e_phi_dot) * (abs(e_phi_dot))^(2-mu) + K1*(abs(s))^(1/2)*sign(s)...
    + s_phi_integ);
u2 = u2 * K;

== matlab function 3.jmavsim_control_smc/fai_d&psi_dGenerator1 ==
  data: u1 input double; pwm1 output double; u2 input double; u3 input double; u4 input double; pwm2 output double; pwm3 output; pwm4 output
function [pwm1,pwm2,pwm3,pwm4] = fcn(u1, u2, u3, u4)

convertMatrix = [-1/sqrt(2)     1/sqrt(2)   1 1;
                1/sqrt(2)       -1/sqrt(2)  1 1;
                1/sqrt(2)       1/sqrt(2)  -1 1;
                -1/sqrt(2)      -1/sqrt(2) -1 1];
pwm = convertMatrix * [u1; u2; u3; u4];
pwm1 = pwm(1);
pwm2 = pwm(2);
pwm3 = pwm(3);
pwm4 = pwm(4);

== matlab function 3.jmavsim_control_smc/Subsystem/MATLAB Function2 ==
  data: dt input; ez input double; u1z output double; ez output; ez_dot output; ez_dot input double; z_des_dotdot input; s_z_integ input; K input; alpha input; beta input; gamma input; mu input; r input; K1 input; K2 input; reset input; s output; s_z_integ output
function [u1z, ez, ez_dot, s, s_z_integ] = u1zfcn(dt, ez, ez_dot, z_des_dotdot,...
                    s_z_integ, K, alpha, beta, gamma, mu, r, K1, K2, reset)

if (reset == 1); s_z_integ = 0; end
m = 0.8; g = 9.80665; %Ix = 0.005; Iy = 0.005; Iz = 0.009; L = 0.33 / 2;
Kz = 0;

% alpha = 2;beta = 1;gamma = 0.4;
% mu = 15/17;r = 5/3;
% K1 = 1;K2 = 1;

s = alpha * ez +  (beta * sign(ez_dot) * (abs(ez_dot)) ^ mu) + (gamma * sign(ez) * (abs(ez)) ^ r);
s_z_integ = s_z_integ + K2 * sign(s) * dt;

u1z = -m*(-g - Kz/m*ez_dot - z_des_dotdot + alpha/(beta*mu)*sign(ez_dot) * (abs(ez_dot))^(2-mu)...
    + gamma*r/(beta*mu)*(sign(ez) * (abs(ez))^(r-1))* sign(ez_dot) * (abs(ez_dot))^(2-mu) + K1*(abs(s))^(1/2)*sign(s)...
    + s_z_integ);

u1z = u1z/(K*m*g);

== matlab function 3.jmavsim_control_smc/Subsystem/MATLAB Function3 ==
  data: ez input double; t input; IAE output; dt input double; IAE input; IAE_t input; IAE_stable input; IAE_stable_t input; reset input; IAE_t output; IAE_stable output; IAE_stable_t output; t output
function [IAE, IAE_t, IAE_stable, IAE_stable_t, t]  = fcn(ez, t, dt, IAE, IAE_t, IAE_stable, IAE_stable_t, reset)

if (reset == 1); t = 0; IAE = 0; IAE_stable = 0; IAE_t = 0; IAE_stable_t = 0; end

t = t + dt;
if (t < 5.01); IAE = IAE + sqrt(ez^2)*dt; end

if (t > 5.00 && t < 10.01); IAE_stable = IAE_stable + sqrt(ez^2)*dt; end

if (t > 4.99 && t < 5.01); IAE_t =  IAE / t; end

if (t > 9.99 && t < 10.01); IAE_stable_t =  IAE_stable / 5; end

== matlab function 3.jmavsim_control_smc/Subsystem/MATLAB Function4 ==
  data: dt input; ex input double; u1x output double; ex output; ex_dot output; ex_dot input double; x_des_dotdot input; s_x_integ input; K input; alpha input; beta input; gamma input; mu input; r input; K1 input; K2 input; reset input; s output; s_x_integ output
function [u1x, ex, ex_dot, s, s_x_integ] = u1xfcn(dt, ex, ex_dot, x_des_dotdot,...
                    s_x_integ, K,alpha, beta, gamma, mu, r, K1, K2, reset)

if (reset == 1); s_x_integ = 0; end
m = 0.8; g = 9.80665; %Ix = 0.005; Iy = 0.005; Iz = 0.009; L = 0.33 / 2;
Kx = 0;

% alpha = 2;beta = 1;gamma = 0.4;
% mu = 15/17;r = 5/3;
% K1 = 1;K2 = 1;

s = alpha * ex +  (beta * sign(ex_dot) * (abs(ex_dot)) ^ mu) + (gamma * sign(ex) * (abs(ex)) ^ r);
s_x_integ = s_x_integ + K2 * sign(s) * dt;

u1x = -m*(- Kx/m*ex_dot - x_des_dotdot + alpha/(beta*mu)*sign(ex_dot) * (abs(ex_dot))^(2-mu)...
    + gamma*r/(beta*mu)*(sign(ex) * (abs(ex))^(r-1))* sign(ex_dot) * (abs(ex_dot))^(2-mu) + K1*(abs(s))^(1/2)*sign(s)...
    + s_x_integ);
u1x = u1x * K;
